simulink model "simulateBPSK"  (R2023b)
settings: Solver=VariableStepAuto  StartTime=0.0  StopTime=10  RelTol=1e-3
InitFcn:
  | bitRate = 1000;  %bits per second
libraries: commdigbbndpm3 x2, commfilt2 x2, commchan3 x1, commrandsrc3 x1, commsink2 x1
settings Model: Creator=prust  LastModifiedBy=龚玲玉
settings SolverCC: AlgebraicLoopSolver=TrustRegion
settings DataIOCC: ReturnWorkspaceOutputs=off
settings DebuggingCC: UnconnectedInputMsg=warning  UnconnectedOutputMsg=warning  UnconnectedLineMsg=warning  ArithmeticOperatorsInVariantConditions=warning
settings ModelReferenceCC: EnableRefExpFcnMdlSchedulingChecks=on
settings SFSimCC: SimUseLocalCustomCode=off  CustomCodeUndefinedFunction=UseInterfaceOnly
settings RTWCC: RTWUseLocalCustomCode=off  DLArmComputeVersion=19.05
settings CodeAppCC: StateflowObjectComments=on

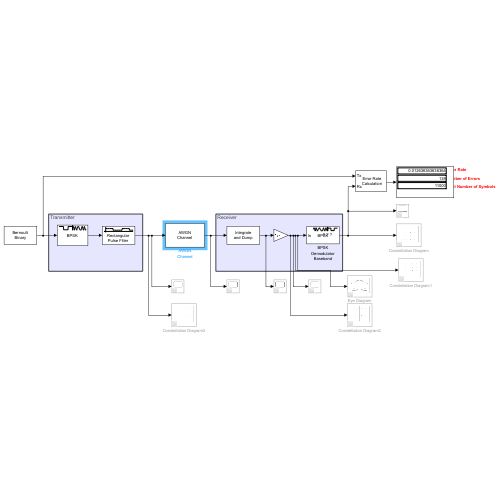
[thumbnail: Simulink's stored preview of the top-level diagram]
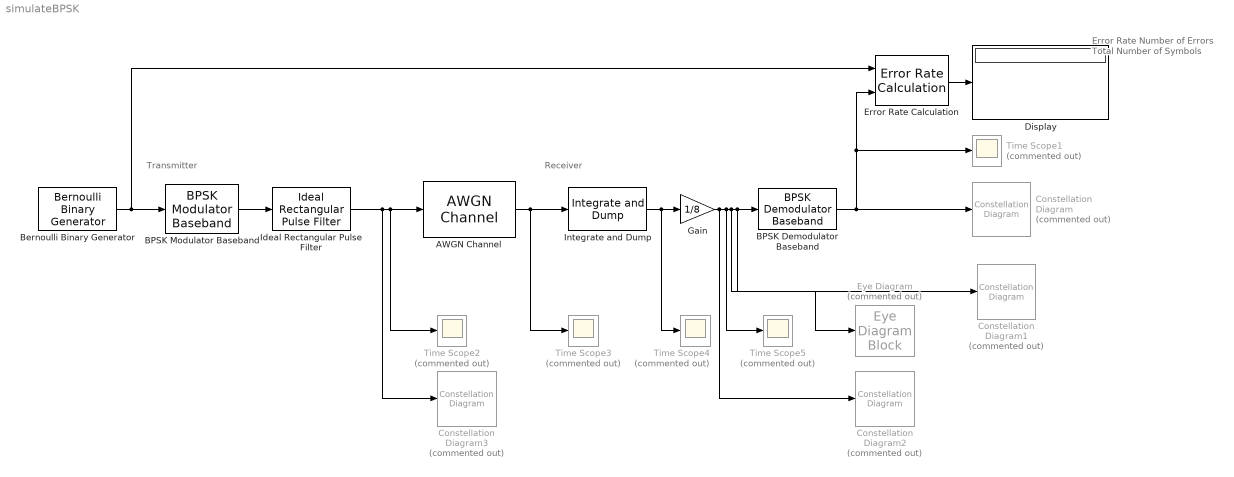
== system simulateBPSK ==
  note: Receiver
  note: Transmitter
  note: Error Rate
      |
      | Number of Errors
      |
      | Total Number of Symbols
  AWGN Channel : commchan3/AWGN Channel  LegacyMode=on  NoiseMethod="Signal to noise ratio  (SNR)"  noiseMode="Signal to noise ratio  (Eb/No)"  EbNo=4  EsNo=6  SNR=60  BitsPerSymbol=1  SignalPower=1  SamplesPerSymbol=1  SymbolPeriod=1/1000  VarianceSource=Parameter  Variance=1  RandomStream=Global stream  Seed=67  SimulateUsing=Interpreted execution
  BPSK Demodulator Baseband : commdigbbndpm3/BPSK Demodulator Baseband  DecType=Hard decision  VarSource=Port  Variance=1  Ph=pi/3  outDtype=double  derotateFactorWordLen=16  derotateFactorDataTypeStr=Inherit: Same word length as input  derotateFactorLastDataTypeStr=Inherit: Same word length as input
  BPSK Modulator Baseband : commdigbbndpm3/BPSK Modulator Baseband  Ph=pi/3  outDtype=double  outWordLen=16  outUDDataType=sfix(16)  outFracLenMode=Best precision  outFracLen=15  outDataTypeStr=double  outLastDataTypeStr=double
  Bernoulli Binary Generator : commrandsrc3/Bernoulli Binary Generator  ProbabilityOfZero=0.5  SeedSource=Auto  Seed=0  SampleTime=0.001  SamplesPerFrame=1000  OutputDataType=double  SimulateUsing=Interpreted execution
  Constellation Diagram : ConstellationDiagram  Commented=on  WindowPosition=[401.000000,117.000000,754.000000,501.000000,]  ScopeFrameLocation=window  ReferenceConstellation=BPSK  XLimits=[-0.91603 1.05]  YLimits=[-1.1618 1.2958]  DefaultConfigurationName=comm.scopes.ConstellationDiagramBlockCfg
  Constellation Diagram1 : ConstellationDiagram  Commented=on  WindowPosition=[451.000000,56.000000,813.000000,778.000000,]  ScopeFrameLocation=window  ReferenceConstellation=BPSK  XLimits=[-1.5773 1.7286]  YLimits=[-1.9906 2.1419]  DefaultConfigurationName=comm.scopes.ConstellationDiagramBlockCfg
  Constellation Diagram2 : ConstellationDiagram  Commented=on  WindowPosition=[451.000000,56.000000,813.000000,778.000000,]  ScopeFrameLocation=window  ReferenceConstellation=BPSK  XLimits=[-1.5773 1.7286]  YLimits=[-1.9906 2.1419]  DefaultConfigurationName=comm.scopes.ConstellationDiagramBlockCfg
  Constellation Diagram3 : ConstellationDiagram  Commented=on  WindowPosition=[451.000000,56.000000,813.000000,778.000000,]  ScopeFrameLocation=window  ReferenceConstellation=BPSK  XLimits=[-1.5773 1.7286]  YLimits=[-1.9906 2.1419]  DefaultConfigurationName=comm.scopes.ConstellationDiagramBlockCfg
  Display : Display
  Error Rate Calculation : commsink2/Error Rate Calculation  N=0  st_delay=0  cp_mode=Entire frame  subframe=[]  PMode=Port  WsName=ErrorVec  RsMode2=off  stop=off  numErr=100  maxBits=1e6
  Eye Diagram : EyeDiagramBlock  Commented=on  WindowPosition=[1.000000,49.000000,1536.000000,793.000000,]  ScopeFrameLocation=window
  Gain : Gain  Gain=1/8
  Ideal Rectangular Pulse Filter : commfilt2/Ideal Rectangular Pulse Filter  pulseLen=8  pulseDelay=0  InputProcessing=Columns as channels (frame based)  RateOptions=Enforce single-rate processing  sampMode=Mute  normCheck=off  normMode=Sum of samples  filterGain=1  saveAsFlag=0  roundingMode=Floor  overflowMode=off  firstCoeffDataTypeStr=Inherit: Same word length as input  firstCoeffMin=[]  firstCoeffMax=[]  firstCoeffLastDataTypeStr=Inherit: Same word length as input  outputDataTypeStr=Inherit: Same as accumulator  outputMin=[]  outputMax=[]  outputLastDataTypeStr=Inherit: Same as accumulator
  Integrate and Dump : commfilt2/Integrate and Dump  obssamples=8  offsetsamples=0  nodump=off  roundingMode=Floor  overflowMode=off  outputDataTypeStr=Inherit: Same as accumulator  outputLastDataTypeStr=Inherit: Same as accumulator
  Time Scope{1..5} (5 alike) : Scope  Commented=on
  wires:
  Bernoulli Binary Generator/1 -> Error Rate Calculation/1, BPSK Modulator Baseband/1
  AWGN Channel/1 -> Time Scope3/1, Integrate and Dump/1
  BPSK Demodulator Baseband/1 -> Constellation Diagram/1, Time Scope1/1, Error Rate Calculation/2
  Error Rate Calculation/1 -> Display/1
  Ideal Rectangular Pulse Filter/1 -> Constellation Diagram3/1, Time Scope2/1, AWGN Channel/1
  Integrate and Dump/1 -> Time Scope4/1, Gain/1
  BPSK Modulator Baseband/1 -> Ideal Rectangular Pulse Filter/1
  Gain/1 -> BPSK Demodulator Baseband/1, Constellation Diagram1/1, Eye Diagram/1, Time Scope5/1, Constellation Diagram2/1
